simulink model "lab3_part2"  (R2019b)
settings: Solver=VariableStepAuto  StartTime=0.0  StopTime=200  RelTol=1e-3
settings Model: Creator=theojanson  LastModifiedBy=theojanson

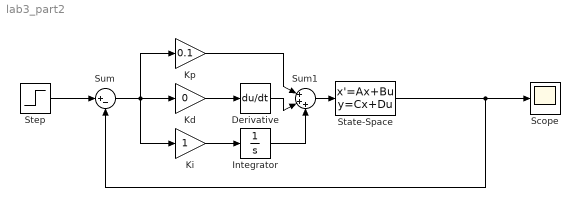
== system lab3_part2 ==
  Derivative : Derivative
  Integrator : Integrator
  Kd : Gain  Gain=0
  Ki : Gain
  Kp : Gain  Gain=0.1
  Scope : Scope
  State-Space : StateSpace  A=[0 1 0 ; 0 -0.1 2 ; 0 -0.04 -20]  B=[0 ; 0 ; 2]  C=[1 0 0]  D=0  InitialCondition=0
  Step : Step  SampleTime=0
  Sum : Sum  Inputs=|+-
  Sum1 : Sum  Inputs=|+++
  wires:
  Step/1 -> Sum/1
  Ki/1 -> Integrator/1
  Sum/1 -> Ki/1, Kd/1, Kp/1
  Kd/1 -> Derivative/1
  Sum1/1 -> State-Space/1
  Kp/1 -> Sum1/1
  Derivative/1 -> Sum1/2
  Integrator/1 -> Sum1/3
  State-Space/1 -> Sum/2, Scope/1
